simulink model "case6"  (R2024b)
settings: Solver=FixedStepAuto  StartTime=0  StopTime=1  FixedStep=1e-7  RelTol=1e-3
values from neighbouring files (symbols this model uses):
  SG_D_1_D = 0.01056    [IEEE9_case_parameters.m]    (also in case1_parameters.m; case2_parameters.m; case3_parameters.m; case4_parameters.m)
  SG_D_1_EnableSaturation = 0    [IEEE9_case_parameters.m]    (also in case1_parameters.m; case2_parameters.m; case3_parameters.m; case4_parameters.m)
  SG_D_1_f0 = 60    [IEEE9_case_parameters.m]    (also in case1_parameters.m; case2_parameters.m; case3_parameters.m; case4_parameters.m)
  SG_D_1_H = 7.5    [IEEE9_case_parameters.m]    (also in case1_parameters.m; case2_parameters.m; case3_parameters.m; case4_parameters.m)
  SG_D_1_K_A = 20    [IEEE9_case_parameters.m]    (also in case1_parameters.m; case2_parameters.m; case3_parameters.m; case4_parameters.m)
  SG_D_1_K_E = 1.000000e+1    (= 10)    [IEEE9_case_parameters.m]    (also in case1_parameters.m; case2_parameters.m; case3_parameters.m; case4_parameters.m)
  SG_D_1_K_F = 2.363    [IEEE9_case_parameters.m]    (also in case1_parameters.m; case2_parameters.m; case3_parameters.m; case4_parameters.m)
  SG_D_1_K_s = 0.5    [IEEE9_case_parameters.m]    (also in case1_parameters.m = 5; case2_parameters.m = 5; case3_parameters.m = 5; case4_parameters.m = 5)
  SG_D_1_R_a = 0.001088    [IEEE9_case_parameters.m]    (also in case1_parameters.m; case2_parameters.m; case3_parameters.m; case4_parameters.m)
  SG_D_1_S_A = 1    [IEEE9_case_parameters.m]    (also in case1_parameters.m; case2_parameters.m; case3_parameters.m; case4_parameters.m)
  SG_D_1_S_B = 0.103    [IEEE9_case_parameters.m]    (also in case1_parameters.m; case2_parameters.m; case3_parameters.m; case4_parameters.m)
  SG_D_1_S_N = 10.659857    [IEEE9_case_parameters.m]    (also in case1_parameters.m; case2_parameters.m; case3_parameters.m; case4_parameters.m)
  SG_D_1_SpeedPara = 200    [IEEE9_case_parameters.m]    (also in case1_parameters.m; case2_parameters.m; case3_parameters.m; case4_parameters.m)
  SG_D_1_T_0 = 0.720173    [IEEE9_case_parameters.m]    (also in case1_parameters.m = 0.755522; case2_parameters.m = 0.808931; case3_parameters.m = 0.869402; case4_parameters.m = 0.729316)
  SG_D_1_T_1 = 0.3    [IEEE9_case_parameters.m]    (also in case1_parameters.m; case2_parameters.m; case3_parameters.m; case4_parameters.m)
  SG_D_1_T_2 = 0.05    [IEEE9_case_parameters.m]    (also in case1_parameters.m; case2_parameters.m; case3_parameters.m; case4_parameters.m)
  SG_D_1_T_3 = 0.02    [IEEE9_case_parameters.m]    (also in case1_parameters.m; case2_parameters.m; case3_parameters.m; case4_parameters.m)
  SG_D_1_T_4 = 0.005    [IEEE9_case_parameters.m]    (also in case1_parameters.m; case2_parameters.m; case3_parameters.m; case4_parameters.m)
  SG_D_1_T_A = 0.02    [IEEE9_case_parameters.m]    (also in case1_parameters.m; case2_parameters.m; case3_parameters.m; case4_parameters.m)
  SG_D_1_T_dd = 8.000000e+0    (= 8)    [IEEE9_case_parameters.m]    (also in case1_parameters.m; case2_parameters.m; case3_parameters.m; case4_parameters.m)
  SG_D_1_T_ddd = 0.04    [IEEE9_case_parameters.m]    (also in case1_parameters.m; case2_parameters.m; case3_parameters.m; case4_parameters.m)
  SG_D_1_T_E = 0.314    [IEEE9_case_parameters.m]    (also in case1_parameters.m; case2_parameters.m; case3_parameters.m; case4_parameters.m)
  SG_D_1_T_F = 0.35    [IEEE9_case_parameters.m]    (also in case1_parameters.m; case2_parameters.m; case3_parameters.m; case4_parameters.m)
  SG_D_1_T_qd = 0.8    [IEEE9_case_parameters.m]    (also in case1_parameters.m; case2_parameters.m; case3_parameters.m; case4_parameters.m)
  SG_D_1_T_qdd = 0.02    [IEEE9_case_parameters.m]    (also in case1_parameters.m; case2_parameters.m; case3_parameters.m; case4_parameters.m)
  SG_D_1_T_speed = 0.1    [IEEE9_case_parameters.m]    (also in case1_parameters.m = 200; case2_parameters.m = 200; case3_parameters.m = 200; case4_parameters.m = 200)
  SG_D_1_T_w = 0.5    [IEEE9_case_parameters.m]    (also in case1_parameters.m; case2_parameters.m; case3_parameters.m; case4_parameters.m)
  SG_D_1_V_ref = 1.990276    [IEEE9_case_parameters.m]    (also in case1_parameters.m = 2.042296; case2_parameters.m = 2.051388; case3_parameters.m = 2.089584; case4_parameters.m = 2.01845)
  SG_D_1_w_ref = 376.991118    [IEEE9_case_parameters.m]    (also in case1_parameters.m; case2_parameters.m; case3_parameters.m; case4_parameters.m)
  SG_D_1_wb = 6.000000e+1    (= 60)    [IEEE9_case_parameters.m]    (also in case1_parameters.m; case2_parameters.m; case3_parameters.m; case4_parameters.m)
  SG_D_1_x_d = 1.9    [IEEE9_case_parameters.m]    (also in case1_parameters.m; case2_parameters.m; case3_parameters.m; case4_parameters.m)
  SG_D_1_x_dd = 0.302    [IEEE9_case_parameters.m]    (also in case1_parameters.m; case2_parameters.m; case3_parameters.m; case4_parameters.m)
  SG_D_1_x_ddd = 0.204    [IEEE9_case_parameters.m]    (also in case1_parameters.m; case2_parameters.m; case3_parameters.m; case4_parameters.m)
  SG_D_1_x_l = 0.05    [IEEE9_case_parameters.m]    (also in case1_parameters.m; case2_parameters.m; case3_parameters.m; case4_parameters.m)
  SG_D_1_x_q = 1.3    [IEEE9_case_parameters.m]    (also in case1_parameters.m; case2_parameters.m; case3_parameters.m; case4_parameters.m)
  SG_D_1_x_qd = 0.5    [IEEE9_case_parameters.m]    (also in case1_parameters.m; case2_parameters.m; case3_parameters.m; case4_parameters.m)
  SG_D_1_x_qdd = 0.3    [IEEE9_case_parameters.m]    (also in case1_parameters.m; case2_parameters.m; case3_parameters.m; case4_parameters.m)
  SG_D_2_D = 0.02    [IEEE9_case_parameters.m]    (also in case1_parameters.m; case2_parameters.m; case3_parameters.m; case4_parameters.m)
  SG_D_2_EnableSaturation = 0    [IEEE9_case_parameters.m]    (also in case1_parameters.m; case2_parameters.m; case3_parameters.m; case4_parameters.m)
  SG_D_2_f0 = 60    [IEEE9_case_parameters.m]    (also in case1_parameters.m; case2_parameters.m; case3_parameters.m; case4_parameters.m)
  SG_D_2_H = 8.000000e+0    (= 8)    [IEEE9_case_parameters.m]    (also in case1_parameters.m; case2_parameters.m; case3_parameters.m; case4_parameters.m)
  SG_D_2_K_A = 20    [IEEE9_case_parameters.m]    (also in case1_parameters.m; case2_parameters.m; case3_parameters.m; case4_parameters.m)
  SG_D_2_K_E = 1.000000e+1    (= 10)    [IEEE9_case_parameters.m]    (also in case1_parameters.m; case2_parameters.m; case3_parameters.m; case4_parameters.m)
  SG_D_2_K_F = 2.363    [IEEE9_case_parameters.m]    (also in case1_parameters.m; case2_parameters.m; case3_parameters.m; case4_parameters.m)
  SG_D_2_K_s = 0.5    [IEEE9_case_parameters.m]    (also in case1_parameters.m = 4; case2_parameters.m = 4; case3_parameters.m = 4; case4_parameters.m = 4)
  SG_D_2_R_a = 0.001088    [IEEE9_case_parameters.m]    (also in case1_parameters.m; case2_parameters.m; case3_parameters.m; case4_parameters.m)
  SG_D_2_S_A = 1    [IEEE9_case_parameters.m]    (also in case1_parameters.m; case2_parameters.m; case3_parameters.m; case4_parameters.m)
  SG_D_2_S_B = 0.103    [IEEE9_case_parameters.m]    (also in case1_parameters.m; case2_parameters.m; case3_parameters.m; case4_parameters.m)
  SG_D_2_S_N = 10.659857    [IEEE9_case_parameters.m]    (also in case1_parameters.m; case2_parameters.m; case3_parameters.m; case4_parameters.m)
  SG_D_2_SpeedPara = 200    [IEEE9_case_parameters.m]    (also in case1_parameters.m; case2_parameters.m; case3_parameters.m; case4_parameters.m)
  SG_D_2_T_0 = 1.632913    [IEEE9_case_parameters.m]    (also in case1_parameters.m = 1.632925; case2_parameters.m = 1.632915; case3_parameters.m = 1.632914; case4_parameters.m = 1.632927)
  SG_D_2_T_1 = 0.2    [IEEE9_case_parameters.m]    (also in case1_parameters.m; case2_parameters.m; case3_parameters.m; case4_parameters.m)
  SG_D_2_T_2 = 0.05    [IEEE9_case_parameters.m]    (also in case1_parameters.m; case2_parameters.m; case3_parameters.m; case4_parameters.m)
  SG_D_2_T_3 = 0.02    [IEEE9_case_parameters.m]    (also in case1_parameters.m; case2_parameters.m; case3_parameters.m; case4_parameters.m)
  SG_D_2_T_4 = 0.005    [IEEE9_case_parameters.m]    (also in case1_parameters.m; case2_parameters.m; case3_parameters.m; case4_parameters.m)
  SG_D_2_T_A = 0.02    [IEEE9_case_parameters.m]    (also in case1_parameters.m; case2_parameters.m; case3_parameters.m; case4_parameters.m)
  SG_D_2_T_dd = 7.9    [IEEE9_case_parameters.m]    (also in case1_parameters.m; case2_parameters.m; case3_parameters.m; case4_parameters.m)
  SG_D_2_T_ddd = 0.04    [IEEE9_case_parameters.m]    (also in case1_parameters.m; case2_parameters.m; case3_parameters.m; case4_parameters.m)
  SG_D_2_T_E = 0.314    [IEEE9_case_parameters.m]    (also in case1_parameters.m; case2_parameters.m; case3_parameters.m; case4_parameters.m)
  SG_D_2_T_F = 0.35    [IEEE9_case_parameters.m]    (also in case1_parameters.m; case2_parameters.m; case3_parameters.m; case4_parameters.m)
  SG_D_2_T_qd = 0.8    [IEEE9_case_parameters.m]    (also in case1_parameters.m; case2_parameters.m; case3_parameters.m; case4_parameters.m)
  SG_D_2_T_qdd = 0.015    [IEEE9_case_parameters.m]    (also in case1_parameters.m; case2_parameters.m; case3_parameters.m; case4_parameters.m)
  SG_D_2_T_speed = 0.1    [IEEE9_case_parameters.m]    (also in case1_parameters.m = 150; case2_parameters.m = 150; case3_parameters.m = 150; case4_parameters.m = 150)
  SG_D_2_T_w = 0.35    [IEEE9_case_parameters.m]    (also in case1_parameters.m; case2_parameters.m; case3_parameters.m; case4_parameters.m)
  SG_D_2_V_ref = 2.58547    [IEEE9_case_parameters.m]    (also in case1_parameters.m = 2.597896; case2_parameters.m = 2.587136; case3_parameters.m = 2.586042; case4_parameters.m = 2.599679)
  SG_D_2_w_ref = 376.991118    [IEEE9_case_parameters.m]    (also in case1_parameters.m; case2_parameters.m; case3_parameters.m; case4_parameters.m)
  SG_D_2_wb = 6.000000e+1    (= 60)    [IEEE9_case_parameters.m]    (also in case1_parameters.m; case2_parameters.m; case3_parameters.m; case4_parameters.m)
  SG_D_2_x_d = 1.8    [IEEE9_case_parameters.m]    (also in case1_parameters.m; case2_parameters.m; case3_parameters.m; case4_parameters.m)
  SG_D_2_x_dd = 0.302    [IEEE9_case_parameters.m]    (also in case1_parameters.m; case2_parameters.m; case3_parameters.m; case4_parameters.m)
  SG_D_2_x_ddd = 0.204    [IEEE9_case_parameters.m]    (also in case1_parameters.m; case2_parameters.m; case3_parameters.m; case4_parameters.m)
  SG_D_2_x_l = 0.05    [IEEE9_case_parameters.m]    (also in case1_parameters.m; case2_parameters.m; case3_parameters.m; case4_parameters.m)
  SG_D_2_x_q = 1.25    [IEEE9_case_parameters.m]    (also in case1_parameters.m; case2_parameters.m; case3_parameters.m; case4_parameters.m)
  SG_D_2_x_qd = 0.5    [IEEE9_case_parameters.m]    (also in case1_parameters.m; case2_parameters.m; case3_parameters.m; case4_parameters.m)
  SG_D_2_x_qdd = 0.3    [IEEE9_case_parameters.m]    (also in case1_parameters.m; case2_parameters.m; case3_parameters.m; case4_parameters.m)
  SG_D_3_D = 0.02    [IEEE9_case_parameters.m]    (also in case1_parameters.m; case2_parameters.m; case3_parameters.m; case4_parameters.m)
  SG_D_3_EnableSaturation = 0    [IEEE9_case_parameters.m]    (also in case1_parameters.m; case2_parameters.m; case3_parameters.m; case4_parameters.m)
  SG_D_3_f0 = 60    [IEEE9_case_parameters.m]    (also in case1_parameters.m; case2_parameters.m; case3_parameters.m; case4_parameters.m)
  SG_D_3_H = 7.7    [IEEE9_case_parameters.m]    (also in case1_parameters.m; case2_parameters.m; case3_parameters.m; case4_parameters.m)
  SG_D_3_K_A = 20    [IEEE9_case_parameters.m]    (also in case1_parameters.m; case2_parameters.m; case3_parameters.m; case4_parameters.m)
  SG_D_3_K_E = 1.000000e+1    (= 10)    [IEEE9_case_parameters.m]    (also in case1_parameters.m; case2_parameters.m; case3_parameters.m; case4_parameters.m)
  SG_D_3_K_F = 2.363    [IEEE9_case_parameters.m]    (also in case1_parameters.m; case2_parameters.m; case3_parameters.m; case4_parameters.m)
  SG_D_3_K_s = 0.2    [IEEE9_case_parameters.m]    (also in case1_parameters.m = 2; case2_parameters.m = 2; case3_parameters.m = 2; case4_parameters.m = 2)
  SG_D_3_R_a = 0.001088    [IEEE9_case_parameters.m]    (also in case1_parameters.m; case2_parameters.m; case3_parameters.m; case4_parameters.m)
  SG_D_3_S_A = 1    [IEEE9_case_parameters.m]    (also in case1_parameters.m; case2_parameters.m; case3_parameters.m; case4_parameters.m)
  SG_D_3_S_B = 0.103    [IEEE9_case_parameters.m]    (also in case1_parameters.m; case2_parameters.m; case3_parameters.m; case4_parameters.m)
  SG_D_3_S_N = 10.659857    [IEEE9_case_parameters.m]    (also in case1_parameters.m; case2_parameters.m; case3_parameters.m; case4_parameters.m)
  SG_D_3_SpeedPara = 200    [IEEE9_case_parameters.m]    (also in case1_parameters.m; case2_parameters.m; case3_parameters.m; case4_parameters.m)
  SG_D_3_T_0 = 0.850788    [IEEE9_case_parameters.m]    (also in case1_parameters.m = 0.850786; case2_parameters.m = 0.850787; case3_parameters.m; case4_parameters.m = 0.850786)
  SG_D_3_T_1 = 0.2    [IEEE9_case_parameters.m]    (also in case1_parameters.m; case2_parameters.m; case3_parameters.m; case4_parameters.m)
  SG_D_3_T_2 = 0.05    [IEEE9_case_parameters.m]    (also in case1_parameters.m; case2_parameters.m; case3_parameters.m; case4_parameters.m)
  SG_D_3_T_3 = 0.02    [IEEE9_case_parameters.m]    (also in case1_parameters.m; case2_parameters.m; case3_parameters.m; case4_parameters.m)
  SG_D_3_T_4 = 0.005    [IEEE9_case_parameters.m]    (also in case1_parameters.m; case2_parameters.m; case3_parameters.m; case4_parameters.m)
  SG_D_3_T_A = 0.02    [IEEE9_case_parameters.m]    (also in case1_parameters.m; case2_parameters.m; case3_parameters.m; case4_parameters.m)
  SG_D_3_T_dd = 8.1    [IEEE9_case_parameters.m]    (also in case1_parameters.m; case2_parameters.m; case3_parameters.m; case4_parameters.m)
  SG_D_3_T_ddd = 0.04    [IEEE9_case_parameters.m]    (also in case1_parameters.m; case2_parameters.m; case3_parameters.m; case4_parameters.m)
  SG_D_3_T_E = 0.314    [IEEE9_case_parameters.m]    (also in case1_parameters.m; case2_parameters.m; case3_parameters.m; case4_parameters.m)
  SG_D_3_T_F = 0.35    [IEEE9_case_parameters.m]    (also in case1_parameters.m; case2_parameters.m; case3_parameters.m; case4_parameters.m)
  SG_D_3_T_qd = 0.8    [IEEE9_case_parameters.m]    (also in case1_parameters.m; case2_parameters.m; case3_parameters.m; case4_parameters.m)
  SG_D_3_T_qdd = 0.015    [IEEE9_case_parameters.m]    (also in case1_parameters.m; case2_parameters.m; case3_parameters.m; case4_parameters.m)
  SG_D_3_T_speed = 0.1    [IEEE9_case_parameters.m]    (also in case1_parameters.m = 180; case2_parameters.m = 180; case3_parameters.m = 180; case4_parameters.m = 180)
  SG_D_3_T_w = 0.4    [IEEE9_case_parameters.m]    (also in case1_parameters.m; case2_parameters.m; case3_parameters.m; case4_parameters.m)
  SG_D_3_V_ref = 1.892727    [IEEE9_case_parameters.m]    (also in case1_parameters.m = 1.906439; case2_parameters.m = 1.895535; case3_parameters.m = 1.892105; case4_parameters.m = 1.906598)
  SG_D_3_w_ref = 376.991118    [IEEE9_case_parameters.m]    (also in case1_parameters.m; case2_parameters.m; case3_parameters.m; case4_parameters.m)
  SG_D_3_wb = 6.000000e+1    (= 60)    [IEEE9_case_parameters.m]    (also in case1_parameters.m; case2_parameters.m; case3_parameters.m; case4_parameters.m)
  SG_D_3_x_d = 1.85    [IEEE9_case_parameters.m]    (also in case1_parameters.m; case2_parameters.m; case3_parameters.m; case4_parameters.m)
  SG_D_3_x_dd = 0.302    [IEEE9_case_parameters.m]    (also in case1_parameters.m; case2_parameters.m; case3_parameters.m; case4_parameters.m)
  SG_D_3_x_ddd = 0.204    [IEEE9_case_parameters.m]    (also in case1_parameters.m; case2_parameters.m; case3_parameters.m; case4_parameters.m)
  SG_D_3_x_l = 0.05    [IEEE9_case_parameters.m]    (also in case1_parameters.m; case2_parameters.m; case3_parameters.m; case4_parameters.m)
  SG_D_3_x_q = 1.2    [IEEE9_case_parameters.m]    (also in case1_parameters.m; case2_parameters.m; case3_parameters.m; case4_parameters.m)
  SG_D_3_x_qd = 0.5    [IEEE9_case_parameters.m]    (also in case1_parameters.m; case2_parameters.m; case3_parameters.m; case4_parameters.m)
  SG_D_3_x_qdd = 0.3    [IEEE9_case_parameters.m]    (also in case1_parameters.m; case2_parameters.m; case3_parameters.m; case4_parameters.m)
(part 8 of 12)

== system case6/SG_D_2/d_psi_d_SG_D_2_block ==
  note: d_psi_d_SG_D_2 in case6
      | $2\,\pi \,f_{0}\,\left(v_{d,\mathrm{SG},D,2}\,\sin\left(\theta _{\mathrm{SG},D,2}\right)-v_{q,\mathrm{SG},D,2}\,\cos\left(\theta _{\mathrm{SG},D,2}\right)+\frac{R_{a}\,\left(\frac{\psi _{\mathrm{1d},\mathrm{SG},D,2}\,\left(x_{\mathrm{dd}}-x_{\mathrm{ddd}}\right)}{x_{\mathrm{dd}}-x_{l}}-\psi _{d,\mathrm{SG},D,2}+\frac{\psi _{\mathrm{fd},\mathrm{SG},D,2}\,\left(x_{\mathrm{ddd}}-x_{l}\right)}{x_{\mathrm{dd}}-x_{l}}\right)}{x_{\mathrm{ddd}}}+\frac{\psi _{q,\mathrm{SG},D,2}\,w_{\mathrm{SG},D,2}}{2\,f_{0}\,\pi }\right)$
      | Automatically generated on 2025-10-31 19:17:31 .
  State_psi_1d_SG_D_2_35cf0 : Inport
  State_psi_d_SG_D_2_1074f : Inport  Port=2
  State_psi_fd_SG_D_2_72eef : Inport  Port=3
  Input_v_d_SG_D_2_2f023 : Inport  Port=4
  State_theta_SG_D_2_812e2 : Inport  Port=5
  Input_v_q_SG_D_2_18101 : Inport  Port=6
  State_theta_SG_D_2_15477 : Inport  Port=7
  State_psi_q_SG_D_2_e45e5 : Inport  Port=8
  State_w_SG_D_2_32109 : Inport  Port=9
  Add_5d9fe : Sum
  Add_af38a : Sum
  Constant_-1_98a73 : Constant  Value=-1
  Constant_-2.0_783ec : Constant  Value=-2.0
  Constant_2.0_d92ce : Constant  Value=2.0
  Constant_R_a_0af9e : Constant  Value=R_a
  Constant_f0_21dda : Constant  Value=f0
  Constant_f0_de244 : Constant  Value=f0
  Constant_pi_26315 : Constant  Value=pi
  Constant_pi_7d260 : Constant  Value=pi
  Constant_x_dd_17b71 : Constant  Value=x_dd
  Constant_x_dd_ba7f9 : Constant  Value=x_dd
  Constant_x_dd_f3294 : Constant  Value=x_dd
  Constant_x_ddd_0bdeb : Constant  Value=x_ddd
  Constant_x_ddd_a16b5 : Constant  Value=x_ddd
  Constant_x_ddd_a17df : Constant  Value=x_ddd
  Constant_x_l_3d893 : Constant  Value=x_l
  Constant_x_l_4d81a : Constant  Value=x_l
  Constant_x_l_d1408 : Constant  Value=x_l
  Divide_43e6a : Product  Inputs=*/
  Divide_65a57 : Product  Inputs=*/
  Divide_c49cc : Product  Inputs=*/
  Divide_fe234 : Product  Inputs=*/
  MathFunc_cos_3f437 : Trigonometry  Operator=cos
  MathFunc_sin_f731c : Trigonometry
  Product_1286d : Product
  Product_50ec1 : Product
  Product_534a2 : Product
  Product_7661a : Product
  Product_80317 : Product
  Product_8572c : Product
  Product_8e728 : Product
  Product_bd5f6 : Product
  Product_be71f : Product
  Product_dae79 : Product
  Product_e87a0 : Product
  Product_fa87c : Product
  Subtract_258f8 : Sum  Inputs=+-
  Subtract_7c26c : Sum  Inputs=+-
  Subtract_7f486 : Sum  Inputs=+-
  Subtract_81009 : Sum  Inputs=+-
  Subtract_ad426 : Sum  Inputs=+-
  Subtract_cd317 : Sum  Inputs=+-
  Subtract_d7885 : Sum  Inputs=+-
  Blockout_d_psi_d_SG_D_2_5e9d3 : Outport
  wires:
  MathFunc_sin_f731c/1 -> Product_be71f/2
  Constant_x_dd_ba7f9/1 -> Subtract_258f8/1
  Constant_-1_98a73/1 -> Product_fa87c/1
  Constant_x_l_4d81a/1 -> Subtract_258f8/2
  State_psi_1d_SG_D_2_35cf0/1 -> Product_fa87c/2
  Constant_f0_21dda/1 -> Product_e87a0/2
  Constant_2.0_d92ce/1 -> Product_8572c/1
  Constant_x_l_3d893/1 -> Subtract_ad426/2
  Constant_x_dd_f3294/1 -> Subtract_d7885/1
  Product_8e728/1 -> Blockout_d_psi_d_SG_D_2_5e9d3/1
  Constant_pi_7d260/1 -> Product_8572c/2
  Constant_x_ddd_a16b5/1 -> Subtract_d7885/2
  Subtract_7f486/1 -> Product_8e728/2
  Product_fa87c/1 -> Product_7661a/1
  Product_8572c/1 -> Product_1286d/1
  Subtract_d7885/1 -> Product_7661a/2
  Divide_c49cc/1 -> Subtract_7f486/2
  Constant_x_ddd_0bdeb/1 -> Subtract_7c26c/1
  Constant_x_l_d1408/1 -> Subtract_7c26c/2
  Product_7661a/1 -> Divide_fe234/1
  Subtract_81009/1 -> Add_af38a/1
  Subtract_258f8/1 -> Divide_fe234/2
  State_psi_fd_SG_D_2_72eef/1 -> Product_50ec1/1
  Subtract_7c26c/1 -> Product_50ec1/2
  Constant_x_dd_17b71/1 -> Subtract_ad426/1
  Divide_fe234/1 -> Add_5d9fe/1
  State_psi_d_SG_D_2_1074f/1 -> Add_5d9fe/2
  Product_50ec1/1 -> Divide_65a57/1
  Subtract_ad426/1 -> Divide_65a57/2
  Add_5d9fe/1 -> Subtract_cd317/1
  Divide_65a57/1 -> Subtract_cd317/2
  Constant_R_a_0af9e/1 -> Product_80317/1
  Subtract_cd317/1 -> Product_80317/2
  Divide_43e6a/1 -> Subtract_81009/1
  State_theta_SG_D_2_812e2/1 -> MathFunc_sin_f731c/1
  Product_80317/1 -> Divide_43e6a/1
  Constant_-2.0_783ec/1 -> Product_bd5f6/1
  Input_v_d_SG_D_2_2f023/1 -> Product_be71f/1
  Constant_x_ddd_a17df/1 -> Divide_43e6a/2
  State_theta_SG_D_2_15477/1 -> MathFunc_cos_3f437/1
  Product_e87a0/1 -> Product_8e728/1
  Product_be71f/1 -> Subtract_81009/2
  Product_bd5f6/1 -> Product_e87a0/1
  Input_v_q_SG_D_2_18101/1 -> Product_dae79/1
  MathFunc_cos_3f437/1 -> Product_dae79/2
  State_psi_q_SG_D_2_e45e5/1 -> Product_534a2/1
  State_w_SG_D_2_32109/1 -> Product_534a2/2
  Constant_f0_de244/1 -> Product_1286d/2
  Constant_pi_26315/1 -> Product_bd5f6/2
  Product_dae79/1 -> Add_af38a/2
  Product_534a2/1 -> Divide_c49cc/1
  Product_1286d/1 -> Divide_c49cc/2
  Add_af38a/1 -> Subtract_7f486/1

== system case6/SG_D_2/d_psi_fd_SG_D_2_block ==
  note: d_psi_fd_SG_D_2 in case6
      | $-\frac{\psi _{\mathrm{fd},\mathrm{SG},D,2}-E_{\mathrm{fd},\mathrm{SG},D,2}+\left(x_{d}-x_{\mathrm{dd}}\right)\,\left(\frac{\frac{\psi _{\mathrm{1d},\mathrm{SG},D,2}\,\left(x_{\mathrm{dd}}-x_{\mathrm{ddd}}\right)}{x_{\mathrm{dd}}-x_{l}}-\psi _{d,\mathrm{SG},D,2}+\frac{\psi _{\mathrm{fd},\mathrm{SG},D,2}\,\left(x_{\mathrm{ddd}}-x_{l}\right)}{x_{\mathrm{dd}}-x_{l}}}{x_{\mathrm{ddd}}}-\frac{\left(x_{\mathrm{dd}}-x_{\mathrm{ddd}}\right)\,\left(\psi _{\mathrm{1d},\mathrm{SG},D,2}-\psi _{\mathrm{fd},\mathrm{SG},D,2}+\frac{\left(x_{\mathrm{dd}}-x_{l}\right)\,\left(\frac{\psi _{\mathrm{1d},\mathrm{SG},D,2}\,\left(x_{\mathrm{dd}}-x_{\mathrm{ddd}}\right)}{x_{\mathrm{dd}}-x_{l}}-\psi _{d,\mathrm{SG},D,2}+\frac{\psi _{\mathrm{fd},\mathrm{SG},D,2}\,\left(x_{\mathrm{ddd}}-x_{l}\right)}{x_{\mathrm{dd}}-x_{l}}\right)}{x_{\mathrm{ddd}}}\right)}{{\left(x_{\mathrm{dd}}-x_{l}\right)}^2}\right)}{T_{\mathrm{dd}}}$
      | Automatically generated on 2025-10-31 19:17:42 .
  State_E_fd_SG_D_2_19eb9 : Inport
  State_psi_fd_SG_D_2_303fb : Inport  Port=2
  State_psi_1d_SG_D_2_6d215 : Inport  Port=3
  State_psi_fd_SG_D_2_241bb : Inport  Port=4
  State_psi_1d_SG_D_2_0a0a1 : Inport  Port=5
  State_psi_d_SG_D_2_52887 : Inport  Port=6
  State_psi_fd_SG_D_2_e38e9 : Inport  Port=7
  State_psi_1d_SG_D_2_47eb6 : Inport  Port=8
  State_psi_d_SG_D_2_9b3b0 : Inport  Port=9
  State_psi_fd_SG_D_2_b670f : Inport  Port=10
  Add_698e0 : Sum
  Add_f958d : Sum
  Constant_-1_7da49 : Constant  Value=-1
  Constant_-1_8f145 : Constant  Value=-1
  Constant_-1_e0119 : Constant  Value=-1
  Constant_2.0_94bfb : Constant  Value=2.0
  Constant_T_dd_c1295 : Constant  Value=T_dd
  Constant_x_d_e6358 : Constant  Value=x_d
  Constant_x_dd_1f29f : Constant  Value=x_dd
  Constant_x_dd_30a93 : Constant  Value=x_dd
  Constant_x_dd_46c1c : Constant  Value=x_dd
  Constant_x_dd_81bb7 : Constant  Value=x_dd
  Constant_x_dd_9e714 : Constant  Value=x_dd
  Constant_x_dd_a8ec9 : Constant  Value=x_dd
  Constant_x_dd_d0077 : Constant  Value=x_dd
  Constant_x_dd_d414e : Constant  Value=x_dd
  Constant_x_dd_d7a8b : Constant  Value=x_dd
  Constant_x_dd_df4d8 : Constant  Value=x_dd
  Constant_x_ddd_1dcf3 : Constant  Value=x_ddd
  Constant_x_ddd_459ed : Constant  Value=x_ddd
  Constant_x_ddd_74016 : Constant  Value=x_ddd
  Constant_x_ddd_9647b : Constant  Value=x_ddd
  Constant_x_ddd_9926d : Constant  Value=x_ddd
  Constant_x_ddd_b0b8f : Constant  Value=x_ddd
  Constant_x_ddd_ee8ce : Constant  Value=x_ddd
  Constant_x_l_04698 : Constant  Value=x_l
  Constant_x_l_1243d : Constant  Value=x_l
  Constant_x_l_1e697 : Constant  Value=x_l
  Constant_x_l_23693 : Constant  Value=x_l
  Constant_x_l_55e04 : Constant  Value=x_l
  Constant_x_l_76dd6 : Constant  Value=x_l
  Constant_x_l_b8c01 : Constant  Value=x_l
  Constant_x_l_bdf4e : Constant  Value=x_l
  Divide_01441 : Product  Inputs=*/
  Divide_0fecb : Product  Inputs=*/
  Divide_38f92 : Product  Inputs=*/
  Divide_68e8e : Product  Inputs=*/
  Divide_75b15 : Product  Inputs=*/
  Divide_94356 : Product  Inputs=*/
  Divide_e5e11 : Product  Inputs=*/
  Divide_f3b5a : Product  Inputs=*/
  Power_f4d65 : Math  Operator=pow
  Product_0b04a : Product
  Product_156d3 : Product
  Product_3cab0 : Product
  Product_42637 : Product
  Product_97702 : Product
  Product_b8a29 : Product
  Product_d15a1 : Product
  Product_d691f : Product
  Product_e1fbf : Product
  Product_e809d : Product
  Subtract_043b7 : Sum  Inputs=+-
  Subtract_0f2a3 : Sum  Inputs=+-
  Subtract_1d7c1 : Sum  Inputs=+-
  Subtract_1dd03 : Sum  Inputs=+-
  Subtract_239ef : Sum  Inputs=+-
  Subtract_363a9 : Sum  Inputs=+-
  Subtract_519ac : Sum  Inputs=+-
  Subtract_56f42 : Sum  Inputs=+-
  Subtract_6a12a : Sum  Inputs=+-
  Subtract_81be0 : Sum  Inputs=+-
  Subtract_9a41b : Sum  Inputs=+-
  Subtract_af6da : Sum  Inputs=+-
  Subtract_b7f89 : Sum  Inputs=+-
  Subtract_bcf40 : Sum  Inputs=+-
  Subtract_c2368 : Sum  Inputs=+-
  Subtract_c5af1 : Sum  Inputs=+-
  Subtract_cb047 : Sum  Inputs=+-
  Subtract_e1520 : Sum  Inputs=+-
  Subtract_f11e5 : Sum  Inputs=+-
  Blockout_d_psi_fd_SG_D_2_3f1a9 : Outport
  wires:
  Constant_x_dd_d0077/1 -> Subtract_e1520/1
  Constant_-1_8f145/1 -> Product_3cab0/1
  Constant_x_l_04698/1 -> Subtract_bcf40/2
  Divide_0fecb/1 -> Add_698e0/1
  Subtract_519ac/1 -> Product_156d3/2
  Constant_x_l_76dd6/1 -> Subtract_e1520/2
  Product_156d3/1 -> Divide_f3b5a/1
  State_psi_1d_SG_D_2_0a0a1/1 -> Product_3cab0/2
  Constant_x_dd_30a93/1 -> Subtract_c2368/1
  Product_e809d/1 -> Divide_0fecb/1
  Constant_x_dd_a8ec9/1 -> Subtract_af6da/1
  Constant_x_ddd_74016/1 -> Subtract_c2368/2
  Constant_x_dd_1f29f/1 -> Subtract_239ef/1
  Product_3cab0/1 -> Product_b8a29/1
  Subtract_c2368/1 -> Product_b8a29/2
  State_psi_d_SG_D_2_9b3b0/1 -> Add_698e0/2
  Constant_x_ddd_ee8ce/1 -> Subtract_519ac/1
  Constant_x_l_bdf4e/1 -> Subtract_519ac/2
  Product_b8a29/1 -> Divide_e5e11/1
  Subtract_e1520/1 -> Divide_e5e11/2
  State_psi_fd_SG_D_2_e38e9/1 -> Product_156d3/1
  Subtract_f11e5/1 -> Product_d15a1/2
  Constant_x_dd_d7a8b/1 -> Subtract_1dd03/1
  Constant_x_l_55e04/1 -> Subtract_1dd03/2
  Product_0b04a/1 -> Product_d15a1/1
  Divide_e5e11/1 -> Add_f958d/1
  State_psi_d_SG_D_2_52887/1 -> Add_f958d/2
  Subtract_1dd03/1 -> Divide_f3b5a/2
  Constant_x_dd_df4d8/1 -> Subtract_bcf40/1
  Constant_x_ddd_9647b/1 -> Subtract_363a9/1
  Add_f958d/1 -> Subtract_81be0/1
  Divide_f3b5a/1 -> Subtract_81be0/2
  Constant_-1_7da49/1 -> Product_42637/1
  Product_97702/1 -> Divide_38f92/1
  State_psi_1d_SG_D_2_47eb6/1 -> Product_42637/2
  Subtract_af6da/1 -> Product_0b04a/2
  Constant_x_dd_46c1c/1 -> Subtract_56f42/1
  Divide_38f92/1 -> Subtract_cb047/2
  Constant_-1_e0119/1 -> Product_0b04a/1
  Constant_x_ddd_b0b8f/1 -> Subtract_56f42/2
  Constant_x_ddd_459ed/1 -> Divide_01441/2
  Subtract_bcf40/1 -> Product_d691f/1
  Subtract_81be0/1 -> Product_d691f/2
  State_psi_fd_SG_D_2_241bb/1 -> Subtract_1d7c1/2
  Product_42637/1 -> Product_e809d/1
  Subtract_56f42/1 -> Product_e809d/2
  Constant_2.0_94bfb/1 -> Power_f4d65/2
  State_psi_1d_SG_D_2_6d215/1 -> Subtract_1d7c1/1
  Constant_x_dd_81bb7/1 -> Subtract_6a12a/1
  Subtract_363a9/1 -> Product_97702/2
  Constant_x_l_b8c01/1 -> Subtract_6a12a/2
  Constant_x_l_23693/1 -> Subtract_363a9/2
  Constant_x_ddd_9926d/1 -> Subtract_af6da/2
  Subtract_239ef/1 -> Divide_38f92/2
  Product_d691f/1 -> Divide_01441/1
  Subtract_6a12a/1 -> Divide_0fecb/2
  State_psi_fd_SG_D_2_b670f/1 -> Product_97702/1
  Constant_x_l_1e697/1 -> Subtract_239ef/2
  Constant_x_dd_d414e/1 -> Subtract_0f2a3/1
  Subtract_1d7c1/1 -> Subtract_f11e5/1
  Divide_01441/1 -> Subtract_f11e5/2
  Constant_x_l_1243d/1 -> Subtract_0f2a3/2
  Subtract_0f2a3/1 -> Power_f4d65/1
  Add_698e0/1 -> Subtract_cb047/1
  Product_d15a1/1 -> Divide_75b15/1
  Power_f4d65/1 -> Divide_75b15/2
  Subtract_cb047/1 -> Divide_94356/1
  Constant_x_ddd_1dcf3/1 -> Divide_94356/2
  Constant_x_d_e6358/1 -> Subtract_043b7/1
  Constant_x_dd_9e714/1 -> Subtract_043b7/2
  Divide_75b15/1 -> Subtract_b7f89/1
  Divide_94356/1 -> Subtract_b7f89/2
  State_E_fd_SG_D_2_19eb9/1 -> Subtract_9a41b/1
  State_psi_fd_SG_D_2_303fb/1 -> Subtract_9a41b/2
  Subtract_043b7/1 -> Product_e1fbf/1
  Subtract_b7f89/1 -> Product_e1fbf/2
  Subtract_9a41b/1 -> Subtract_c5af1/1
  Product_e1fbf/1 -> Subtract_c5af1/2
  Subtract_c5af1/1 -> Divide_68e8e/1
  Constant_T_dd_c1295/1 -> Divide_68e8e/2
  Divide_68e8e/1 -> Blockout_d_psi_fd_SG_D_2_3f1a9/1

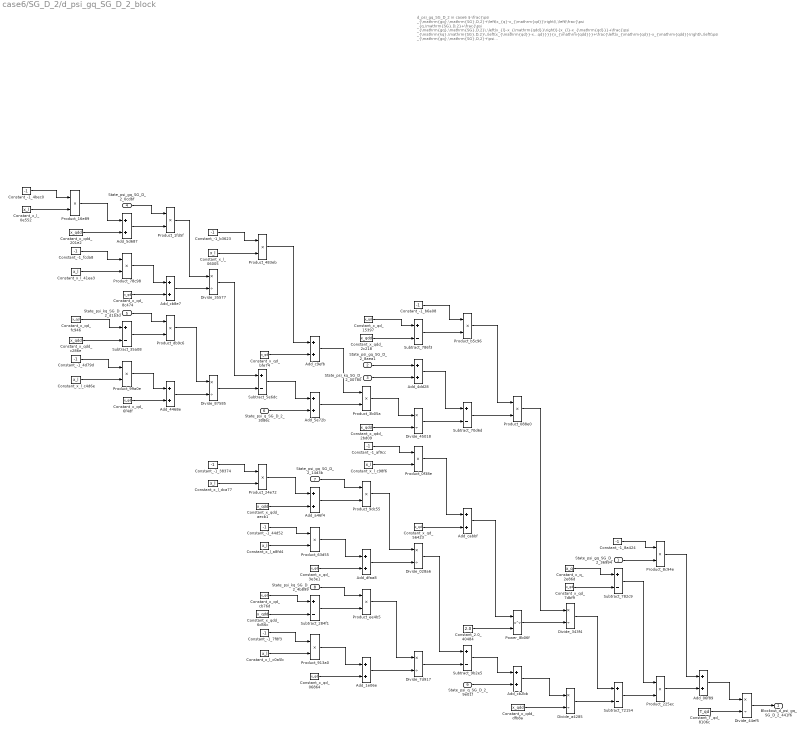
== system case6/SG_D_2/d_psi_gq_SG_D_2_block ==
  note: d_psi_gq_SG_D_2 in case6
      | $-\frac{\psi _{\mathrm{gq},\mathrm{SG},D,2}+\left(x_{q}-x_{\mathrm{qd}}\right)\,\left(\frac{\psi _{q,\mathrm{SG},D,2}+\frac{\psi _{\mathrm{gq},\mathrm{SG},D,2}\,\left(x_{l}-x_{\mathrm{qdd}}\right)}{x_{l}-x_{\mathrm{qd}}}+\frac{\psi _{\mathrm{kq},\mathrm{SG},D,2}\,\left(x_{\mathrm{qd}}-x_{\mathrm{qdd}}\right)}{x_{l}-x_{\mathrm{qd}}}}{x_{\mathrm{qdd}}}+\frac{\left(x_{\mathrm{qd}}-x_{\mathrm{qdd}}\right)\,\left(\psi _{\mathrm{gq},\mathrm{SG},D,2}+\psi _{\mathrm{kq},\mathrm{SG},D,2}+\frac{\left(x_{l}-x_{\mathrm{qd}}\right)\,\left(\psi _{q,\mathrm{SG},D,2}+\frac{\psi _{\mathrm{gq},\mathrm{SG},D,2}\,\left(x_{l}-x_{\mathrm{qdd}}\right)}{x_{l}-x_{\mathrm{qd}}}+\frac{\psi _{\mathrm{kq},\mathrm{SG},D,2}\,\left(x_{\mathrm{qd}}-x_{\mathrm{qdd}}\right)}{x_{l}-x_{\mathrm{qd}}}\right)}{x_{\mathrm{qdd}}}\right)}{{\left(x_{l}-x_{\mathrm{qd}}\right)}^2}\right)}{T_{\mathrm{qd}}}$
      | Automatically generated on 2025-10-31 19:17:52 .
  State_psi_gq_SG_D_2_36994 : Inport
  State_psi_gq_SG_D_2_8aea1 : Inport  Port=2
  State_psi_kq_SG_D_2_00780 : Inport  Port=3
  State_psi_gq_SG_D_2_0cdbf : Inport  Port=4
  State_psi_kq_SG_D_2_d1b3d : Inport  Port=5
  State_psi_q_SG_D_2_3086c : Inport  Port=6
  State_psi_gq_SG_D_2_14d3b : Inport  Port=7
  State_psi_kq_SG_D_2_4b899 : Inport  Port=8
  State_psi_q_SG_D_2_9e01f : Inport  Port=9
  Add_06f89 : Sum
  Add_1e06e : Sum
  Add_4468e : Sum
  Add_4dd28 : Sum
  Add_5d687 : Sum
  Add_5e72b : Sum
  Add_a46f4 : Sum
  Add_c9efb : Sum
  Add_cabbf : Sum
  Add_cb2bb : Sum
  Add_cb8e7 : Sum
  Add_dfaa8 : Sum
  Constant_-1_38374 : Constant  Value=-1
  Constant_-1_44d52 : Constant  Value=-1
  Constant_-1_4bec0 : Constant  Value=-1
  Constant_-1_4d79d : Constant  Value=-1
  Constant_-1_7f8f3 : Constant  Value=-1
  Constant_-1_8a424 : Constant  Value=-1
  Constant_-1_af9cc : Constant  Value=-1
  Constant_-1_b3623 : Constant  Value=-1
  Constant_-1_b6a08 : Constant  Value=-1
  Constant_-1_fcda8 : Constant  Value=-1
  Constant_2.0_40484 : Constant  Value=2.0
  Constant_T_qd_8106c : Constant  Value=T_qd
  Constant_x_l_06005 : Constant  Value=x_l
  Constant_x_l_0e552 : Constant  Value=x_l
  Constant_x_l_41ea3 : Constant  Value=x_l
  Constant_x_l_a8fd4 : Constant  Value=x_l
  Constant_x_l_c0a5b : Constant  Value=x_l
  Constant_x_l_c4d6e : Constant  Value=x_l
  Constant_x_l_c98f6 : Constant  Value=x_l
  Constant_x_l_dca77 : Constant  Value=x_l
  Constant_x_q_2e86d : Constant  Value=x_q
  Constant_x_qd_06864 : Constant  Value=x_qd
  Constant_x_qd_15397 : Constant  Value=x_qd
  Constant_x_qd_3e3e1 : Constant  Value=x_qd
  Constant_x_qd_56423 : Constant  Value=x_qd
  Constant_x_qd_6f4df : Constant  Value=x_qd
  Constant_x_qd_7dbf9 : Constant  Value=x_qd
  Constant_x_qd_8c474 : Constant  Value=x_qd
  Constant_x_qd_bfe74 : Constant  Value=x_qd
  Constant_x_qd_cb76d : Constant  Value=x_qd
  Constant_x_qd_fc946 : Constant  Value=x_qd
  Constant_x_qdd_201e2 : Constant  Value=x_qdd
  Constant_x_qdd_2bd09 : Constant  Value=x_qdd
  Constant_x_qdd_2c218 : Constant  Value=x_qdd
  Constant_x_qdd_6d56c : Constant  Value=x_qdd
  Constant_x_qdd_aecb1 : Constant  Value=x_qdd
  Constant_x_qdd_c286e : Constant  Value=x_qdd
  Constant_x_qdd_dfb8a : Constant  Value=x_qdd
  Divide_028a6 : Product  Inputs=*/
  Divide_343f4 : Product  Inputs=*/
  Divide_35577 : Product  Inputs=*/
  Divide_44ef5 : Product  Inputs=*/
  Divide_45018 : Product  Inputs=*/
  Divide_7d917 : Product  Inputs=*/
  Divide_87585 : Product  Inputs=*/
  Divide_a4285 : Product  Inputs=*/
  Power_8b06f : Math  Operator=pow
  Product_088e0 : Product
  Product_0f38e : Product
  Product_16e89 : Product
  Product_1fd5f : Product
  Product_225ec : Product
  Product_24e72 : Product
  Product_3b05a : Product
  Product_483eb : Product
  Product_63d55 : Product
  Product_78c98 : Product
  Product_8c94e : Product
  Product_913a0 : Product
  Product_99a0e : Product
  Product_9dc55 : Product
  Product_b5c96 : Product
  Product_db9c6 : Product
  Product_ee4b5 : Product
  Subtract_284f1 : Sum  Inputs=+-
  Subtract_35a08 : Sum  Inputs=+-
  Subtract_5e6dc : Sum  Inputs=+-
  Subtract_70d6d : Sum  Inputs=+-
  Subtract_72154 : Sum  Inputs=+-
  Subtract_782c9 : Sum  Inputs=+-
  Subtract_786f3 : Sum  Inputs=+-
  Subtract_9b2e5 : Sum  Inputs=+-
  Blockout_d_psi_gq_SG_D_2_441f6 : Outport
  wires:
  Constant_x_l_c0a5b/1 -> Product_913a0/2
  Constant_x_l_dca77/1 -> Product_24e72/2
  Constant_x_qd_fc946/1 -> Subtract_35a08/1
  Constant_x_l_c98f6/1 -> Product_0f38e/2
  Constant_x_qdd_2c218/1 -> Subtract_786f3/2
  Constant_-1_4d79d/1 -> Product_99a0e/1
  Constant_-1_4bec0/1 -> Product_16e89/1
  State_psi_gq_SG_D_2_8aea1/1 -> Add_4dd28/1
  Constant_x_qdd_c286e/1 -> Subtract_35a08/2
  Constant_x_qd_15397/1 -> Subtract_786f3/1
  Constant_x_l_c4d6e/1 -> Product_99a0e/2
  Constant_x_l_0e552/1 -> Product_16e89/2
  Product_99a0e/1 -> Add_4468e/1
  Product_16e89/1 -> Add_5d687/1
  Constant_x_l_41ea3/1 -> Product_78c98/2
  Constant_x_l_06005/1 -> Product_483eb/2
  Constant_x_qd_6f4df/1 -> Add_4468e/2
  Constant_x_qdd_201e2/1 -> Add_5d687/2
  Constant_-1_fcda8/1 -> Product_78c98/1
  Constant_x_qd_06864/1 -> Add_1e06e/2
  Constant_x_qdd_aecb1/1 -> Add_a46f4/2
  State_psi_gq_SG_D_2_0cdbf/1 -> Product_1fd5f/1
  Add_4468e/1 -> Divide_87585/2
  Add_5d687/1 -> Product_1fd5f/2
  Constant_x_qd_7dbf9/1 -> Subtract_782c9/2
  Product_78c98/1 -> Add_cb8e7/1
  Constant_x_qd_8c474/1 -> Add_cb8e7/2
  State_psi_kq_SG_D_2_d1b3d/1 -> Product_db9c6/1
  Divide_35577/1 -> Subtract_5e6dc/1
  Subtract_35a08/1 -> Product_db9c6/2
  Product_1fd5f/1 -> Divide_35577/1
  Add_cb8e7/1 -> Divide_35577/2
  Add_5e72b/1 -> Product_3b05a/2
  Product_db9c6/1 -> Divide_87585/1
  Constant_-1_b3623/1 -> Product_483eb/1
  Divide_87585/1 -> Subtract_5e6dc/2
  Constant_-1_7f8f3/1 -> Product_913a0/1
  Constant_-1_38374/1 -> Product_24e72/1
  Product_483eb/1 -> Add_c9efb/1
  Constant_x_qdd_6d56c/1 -> Subtract_284f1/2
  Constant_x_qd_bfe74/1 -> Add_c9efb/2
  Subtract_5e6dc/1 -> Add_5e72b/1
  Constant_-1_af9cc/1 -> Product_0f38e/1
  State_psi_q_SG_D_2_3086c/1 -> Add_5e72b/2
  Product_913a0/1 -> Add_1e06e/1
  Product_24e72/1 -> Add_a46f4/1
  Constant_-1_44d52/1 -> Product_63d55/1
  Product_3b05a/1 -> Divide_45018/1
  Constant_x_l_a8fd4/1 -> Product_63d55/2
  Product_225ec/1 -> Add_06f89/2
  Constant_x_qd_cb76d/1 -> Subtract_284f1/1
  Add_c9efb/1 -> Product_3b05a/1
  State_psi_gq_SG_D_2_14d3b/1 -> Product_9dc55/1
  Add_1e06e/1 -> Divide_7d917/2
  Add_a46f4/1 -> Product_9dc55/2
  Product_63d55/1 -> Add_dfaa8/1
  Constant_x_qd_3e3e1/1 -> Add_dfaa8/2
  State_psi_kq_SG_D_2_4b899/1 -> Product_ee4b5/1
  Subtract_284f1/1 -> Product_ee4b5/2
  Divide_7d917/1 -> Subtract_9b2e5/2
  State_psi_kq_SG_D_2_00780/1 -> Add_4dd28/2
  Product_ee4b5/1 -> Divide_7d917/1
  Constant_x_qdd_2bd09/1 -> Divide_45018/2
  Product_9dc55/1 -> Divide_028a6/1
  Add_dfaa8/1 -> Divide_028a6/2
  Constant_-1_b6a08/1 -> Product_b5c96/1
  Subtract_786f3/1 -> Product_b5c96/2
  Add_4dd28/1 -> Subtract_70d6d/1
  Divide_45018/1 -> Subtract_70d6d/2
  Product_0f38e/1 -> Add_cabbf/1
  Constant_x_qd_56423/1 -> Add_cabbf/2
  Divide_028a6/1 -> Subtract_9b2e5/1
  Product_b5c96/1 -> Product_088e0/1
  Subtract_70d6d/1 -> Product_088e0/2
  Add_cabbf/1 -> Power_8b06f/1
  Constant_2.0_40484/1 -> Power_8b06f/2
  Subtract_9b2e5/1 -> Add_cb2bb/1
  State_psi_q_SG_D_2_9e01f/1 -> Add_cb2bb/2
  Product_088e0/1 -> Divide_343f4/1
  Power_8b06f/1 -> Divide_343f4/2
  Add_cb2bb/1 -> Divide_a4285/1
  Constant_x_qdd_dfb8a/1 -> Divide_a4285/2
  Constant_x_q_2e86d/1 -> Subtract_782c9/1
  Divide_343f4/1 -> Subtract_72154/1
  Divide_a4285/1 -> Subtract_72154/2
  Divide_44ef5/1 -> Blockout_d_psi_gq_SG_D_2_441f6/1
  Constant_-1_8a424/1 -> Product_8c94e/1
  State_psi_gq_SG_D_2_36994/1 -> Product_8c94e/2
  Subtract_782c9/1 -> Product_225ec/1
  Subtract_72154/1 -> Product_225ec/2
  Product_8c94e/1 -> Add_06f89/1
  Add_06f89/1 -> Divide_44ef5/1
  Constant_T_qd_8106c/1 -> Divide_44ef5/2

== system case6/SG_D_2/d_psi_kq_SG_D_2_block ==
  note: d_psi_kq_SG_D_2 in case6
      | $-\frac{\psi _{\mathrm{gq},\mathrm{SG},D,2}+\psi _{\mathrm{kq},\mathrm{SG},D,2}+\frac{\left(x_{l}-x_{\mathrm{qd}}\right)\,\left(\psi _{q,\mathrm{SG},D,2}+\frac{\psi _{\mathrm{gq},\mathrm{SG},D,2}\,\left(x_{l}-x_{\mathrm{qdd}}\right)}{x_{l}-x_{\mathrm{qd}}}+\frac{\psi _{\mathrm{kq},\mathrm{SG},D,2}\,\left(x_{\mathrm{qd}}-x_{\mathrm{qdd}}\right)}{x_{l}-x_{\mathrm{qd}}}\right)}{x_{\mathrm{qdd}}}}{T_{\mathrm{qdd}}}$
      | Automatically generated on 2025-10-31 19:17:55 .
  State_psi_gq_SG_D_2_dc43a : Inport
  State_psi_kq_SG_D_2_17791 : Inport  Port=2
  State_psi_gq_SG_D_2_a7d32 : Inport  Port=3
  State_psi_kq_SG_D_2_51ab3 : Inport  Port=4
  State_psi_q_SG_D_2_b3f78 : Inport  Port=5
  Add_0df17 : Sum
  Add_16491 : Sum
  Add_1eaf4 : Sum
  Add_4b865 : Sum
  Add_cfabd : Sum
  Add_f1156 : Sum
  Constant_-1_3a961 : Constant  Value=-1
  Constant_-1_8485d : Constant  Value=-1
  Constant_-1_9430f : Constant  Value=-1
  Constant_-1_e52d4 : Constant  Value=-1
  Constant_-1_e5725 : Constant  Value=-1
  Constant_T_qdd_5a871 : Constant  Value=T_qdd
  Constant_x_l_0699e : Constant  Value=x_l
  Constant_x_l_57848 : Constant  Value=x_l
  Constant_x_l_58a37 : Constant  Value=x_l
  Constant_x_l_6508b : Constant  Value=x_l
  Constant_x_qd_30723 : Constant  Value=x_qd
  Constant_x_qd_e3960 : Constant  Value=x_qd
  Constant_x_qd_ee3c4 : Constant  Value=x_qd
  Constant_x_qd_f9075 : Constant  Value=x_qd
  Constant_x_qdd_63c30 : Constant  Value=x_qdd
  Constant_x_qdd_c05d3 : Constant  Value=x_qdd
  Constant_x_qdd_cc31c : Constant  Value=x_qdd
  Divide_72e9f : Product  Inputs=*/
  Divide_b17f8 : Product  Inputs=*/
  Divide_eb976 : Product  Inputs=*/
  Divide_f11e8 : Product  Inputs=*/
  Product_124f4 : Product
  Product_72f2f : Product
  Product_8e346 : Product
  Product_a2ec3 : Product
  Product_b9bb0 : Product
  Product_e4590 : Product
  Product_f7c05 : Product
  Product_fe7c3 : Product
  Subtract_36be7 : Sum  Inputs=+-
  Subtract_71df2 : Sum  Inputs=+-
  Subtract_fb314 : Sum  Inputs=+-
  Blockout_d_psi_kq_SG_D_2_04077 : Outport
  wires:
  State_psi_kq_SG_D_2_17791/1 -> Subtract_fb314/2
  Constant_-1_e52d4/1 -> Product_a2ec3/1
  Constant_-1_9430f/1 -> Product_72f2f/1
  Constant_x_l_58a37/1 -> Product_72f2f/2
  Constant_x_qdd_c05d3/1 -> Add_16491/2
  Constant_x_l_0699e/1 -> Product_a2ec3/2
  Constant_x_qd_e3960/1 -> Subtract_71df2/1
  Constant_T_qdd_5a871/1 -> Divide_f11e8/2
  Constant_-1_e5725/1 -> Product_fe7c3/1
  Product_72f2f/1 -> Add_16491/1
  Constant_x_qdd_cc31c/1 -> Subtract_71df2/2
  Constant_x_l_6508b/1 -> Product_fe7c3/2
  Divide_f11e8/1 -> Blockout_d_psi_kq_SG_D_2_04077/1
  State_psi_gq_SG_D_2_a7d32/1 -> Product_e4590/1
  Add_16491/1 -> Product_e4590/2
  Product_a2ec3/1 -> Add_f1156/1
  Constant_x_qd_30723/1 -> Add_f1156/2
  Product_b9bb0/1 -> Divide_eb976/1
  State_psi_kq_SG_D_2_51ab3/1 -> Product_8e346/1
  Subtract_71df2/1 -> Product_8e346/2
  Product_fe7c3/1 -> Add_1eaf4/1
  Constant_x_qd_ee3c4/1 -> Add_1eaf4/2
  Product_8e346/1 -> Divide_72e9f/1
  Product_e4590/1 -> Divide_b17f8/1
  Add_f1156/1 -> Divide_b17f8/2
  Add_1eaf4/1 -> Divide_72e9f/2
  State_psi_q_SG_D_2_b3f78/1 -> Add_cfabd/2
  Constant_-1_8485d/1 -> Product_124f4/1
  Constant_x_l_57848/1 -> Product_124f4/2
  Divide_b17f8/1 -> Subtract_36be7/1
  Divide_72e9f/1 -> Subtract_36be7/2
  Product_124f4/1 -> Add_0df17/1
  Constant_x_qd_f9075/1 -> Add_0df17/2
  Subtract_36be7/1 -> Add_cfabd/1
  Constant_x_qdd_63c30/1 -> Divide_eb976/2
  Constant_-1_3a961/1 -> Product_f7c05/1
  State_psi_gq_SG_D_2_dc43a/1 -> Product_f7c05/2
  Add_0df17/1 -> Product_b9bb0/1
  Add_cfabd/1 -> Product_b9bb0/2
  Product_f7c05/1 -> Subtract_fb314/1
  Subtract_fb314/1 -> Add_4b865/1
  Divide_eb976/1 -> Add_4b865/2
  Add_4b865/1 -> Divide_f11e8/1

== system case6/SG_D_2/d_psi_q_SG_D_2_block ==
  note: d_psi_q_SG_D_2 in case6
      | $2\,\pi \,f_{0}\,\left(v_{d,\mathrm{SG},D,2}\,\cos\left(\theta _{\mathrm{SG},D,2}\right)+v_{q,\mathrm{SG},D,2}\,\sin\left(\theta _{\mathrm{SG},D,2}\right)-\frac{R_{a}\,\left(\psi _{q,\mathrm{SG},D,2}+\frac{\psi _{\mathrm{gq},\mathrm{SG},D,2}\,\left(x_{l}-x_{\mathrm{qdd}}\right)}{x_{l}-x_{\mathrm{qd}}}+\frac{\psi _{\mathrm{kq},\mathrm{SG},D,2}\,\left(x_{\mathrm{qd}}-x_{\mathrm{qdd}}\right)}{x_{l}-x_{\mathrm{qd}}}\right)}{x_{\mathrm{qdd}}}-\frac{\psi _{d,\mathrm{SG},D,2}\,w_{\mathrm{SG},D,2}}{2\,f_{0}\,\pi }\right)$
      | Automatically generated on 2025-10-31 19:17:36 .
  State_psi_gq_SG_D_2_12de1 : Inport
  State_psi_kq_SG_D_2_25a64 : Inport  Port=2
  State_psi_q_SG_D_2_571db : Inport  Port=3
  Input_v_d_SG_D_2_48357 : Inport  Port=4
  State_theta_SG_D_2_b5a9c : Inport  Port=5
  Input_v_q_SG_D_2_9b22c : Inport  Port=6
  State_theta_SG_D_2_25188 : Inport  Port=7
  State_psi_d_SG_D_2_57873 : Inport  Port=8
  State_w_SG_D_2_3c58c : Inport  Port=9
  Add_1d066 : Sum
  Add_38483 : Sum
  Add_5fcfb : Sum
  Add_7f6a1 : Sum
  Add_8ff6d : Sum
  Constant_-1_3e0c4 : Constant  Value=-1
  Constant_-1_43afb : Constant  Value=-1
  Constant_-1_9eeab : Constant  Value=-1
  Constant_-2.0_212f6 : Constant  Value=-2.0
  Constant_2.0_9726f : Constant  Value=2.0
  Constant_R_a_16b3c : Constant  Value=R_a
  Constant_f0_1eb0c : Constant  Value=f0
  Constant_f0_bb4e5 : Constant  Value=f0
  Constant_pi_87183 : Constant  Value=pi
  Constant_pi_cc331 : Constant  Value=pi
  Constant_x_l_50222 : Constant  Value=x_l
  Constant_x_l_bc9d0 : Constant  Value=x_l
  Constant_x_l_fe552 : Constant  Value=x_l
  Constant_x_qd_106ce : Constant  Value=x_qd
  Constant_x_qd_b2279 : Constant  Value=x_qd
  Constant_x_qd_fefb8 : Constant  Value=x_qd
  Constant_x_qdd_a4da7 : Constant  Value=x_qdd
  Constant_x_qdd_b1a02 : Constant  Value=x_qdd
  Constant_x_qdd_e7470 : Constant  Value=x_qdd
  Divide_0a8d3 : Product  Inputs=*/
  Divide_0bb9f : Product  Inputs=*/
  Divide_693d2 : Product  Inputs=*/
  Divide_9f2bc : Product  Inputs=*/
  MathFunc_cos_4d8c9 : Trigonometry  Operator=cos
  MathFunc_sin_53da8 : Trigonometry
  Product_0d1c8 : Product
  Product_0d858 : Product
  Product_1dc74 : Product
  Product_26c46 : Product
  Product_37b99 : Product
  Product_3aed0 : Product
  Product_6eeda : Product
  Product_7e84f : Product
  Product_8b1ea : Product
  Product_9c0ed : Product
  Product_a934e : Product
  Product_dfbfa : Product
  Product_e33d9 : Product
  Product_f8e8e : Product
  Subtract_2236c : Sum  Inputs=+-
  Subtract_6b90f : Sum  Inputs=+-
  Subtract_bbc9a : Sum  Inputs=+-
  Subtract_eaa3a : Sum  Inputs=+-
  Blockout_d_psi_q_SG_D_2_fdda2 : Outport
  wires:
  Constant_x_qdd_b1a02/1 -> Subtract_bbc9a/2
  Constant_x_l_50222/1 -> Product_7e84f/2
  Constant_-1_3e0c4/1 -> Product_dfbfa/1
  Constant_x_l_fe552/1 -> Product_dfbfa/2
  Product_dfbfa/1 -> Add_1d066/1
  Constant_pi_cc331/1 -> Product_9c0ed/2
  State_psi_gq_SG_D_2_12de1/1 -> Product_0d1c8/1
  Constant_x_l_bc9d0/1 -> Product_37b99/2
  State_w_SG_D_2_3c58c/1 -> Product_e33d9/2
  Constant_x_qd_b2279/1 -> Add_8ff6d/2
  Constant_x_qdd_e7470/1 -> Add_1d066/2
  Constant_2.0_9726f/1 -> Product_9c0ed/1
  Constant_-1_9eeab/1 -> Product_37b99/1
  Constant_x_qd_106ce/1 -> Subtract_bbc9a/1
  Constant_-1_43afb/1 -> Product_7e84f/1
  State_psi_q_SG_D_2_571db/1 -> Add_38483/2
  Add_1d066/1 -> Product_0d1c8/2
  Product_9c0ed/1 -> Product_0d858/1
  Product_37b99/1 -> Add_7f6a1/1
  Constant_pi_87183/1 -> Product_a934e/2
  Constant_f0_bb4e5/1 -> Product_0d858/2
  Constant_x_qd_fefb8/1 -> Add_7f6a1/2
  State_psi_kq_SG_D_2_25a64/1 -> Product_6eeda/1
  Subtract_bbc9a/1 -> Product_6eeda/2
  Product_7e84f/1 -> Add_8ff6d/1
  Input_v_q_SG_D_2_9b22c/1 -> Product_1dc74/1
  Product_0d1c8/1 -> Divide_0a8d3/1
  Product_0d858/1 -> Divide_9f2bc/2
  Add_7f6a1/1 -> Divide_0a8d3/2
  Product_6eeda/1 -> Divide_0bb9f/1
  Add_8ff6d/1 -> Divide_0bb9f/2
  Divide_0a8d3/1 -> Subtract_6b90f/1
  State_theta_SG_D_2_b5a9c/1 -> MathFunc_cos_4d8c9/1
  Divide_0bb9f/1 -> Subtract_6b90f/2
  Subtract_6b90f/1 -> Add_38483/1
  MathFunc_cos_4d8c9/1 -> Product_26c46/2
  Constant_R_a_16b3c/1 -> Product_8b1ea/1
  Add_38483/1 -> Product_8b1ea/2
  State_theta_SG_D_2_25188/1 -> MathFunc_sin_53da8/1
  Product_8b1ea/1 -> Divide_693d2/1
  Product_a934e/1 -> Product_f8e8e/1
  Product_1dc74/1 -> Subtract_2236c/2
  Constant_x_qdd_a4da7/1 -> Divide_693d2/2
  Input_v_d_SG_D_2_48357/1 -> Product_26c46/1
  Add_5fcfb/1 -> Product_3aed0/2
  Divide_693d2/1 -> Subtract_eaa3a/1
  Product_26c46/1 -> Subtract_eaa3a/2
  MathFunc_sin_53da8/1 -> Product_1dc74/2
  Product_3aed0/1 -> Blockout_d_psi_q_SG_D_2_fdda2/1
  State_psi_d_SG_D_2_57873/1 -> Product_e33d9/1
  Constant_-2.0_212f6/1 -> Product_a934e/1
  Product_f8e8e/1 -> Product_3aed0/1
  Subtract_eaa3a/1 -> Subtract_2236c/1
  Product_e33d9/1 -> Divide_9f2bc/1
  Constant_f0_1eb0c/1 -> Product_f8e8e/2
  Subtract_2236c/1 -> Add_5fcfb/1
  Divide_9f2bc/1 -> Add_5fcfb/2

== system case6/SG_D_2/d_theta_SG_D_2_block ==
  note: d_theta_SG_D_2 in case6
      | $w_{\mathrm{SG},D,2}-2\,\pi \,f_{0}$
      | Automatically generated on 2025-10-31 19:18:04 .
  State_w_SG_D_2_cb344 : Inport
  Add_10eb3 : Sum
  Constant_-2.0_6bd74 : Constant  Value=-2.0
  Constant_f0_8f96a : Constant  Value=f0
  Constant_pi_22cbd : Constant  Value=pi
  Product_26c39 : Product
  Product_ff792 : Product
  Blockout_d_theta_SG_D_2_0f7ec : Outport
  wires:
  Constant_-2.0_6bd74/1 -> Product_26c39/1
  Constant_pi_22cbd/1 -> Product_26c39/2
  Add_10eb3/1 -> Blockout_d_theta_SG_D_2_0f7ec/1
  Product_26c39/1 -> Product_ff792/1
  Constant_f0_8f96a/1 -> Product_ff792/2
  Product_ff792/1 -> Add_10eb3/1
  State_w_SG_D_2_cb344/1 -> Add_10eb3/2
